simulink model "Tester_GX"  (R2026a)
settings: Solver=VariableStepAuto  StopTime=inf
libraries: instrumentlib x2, dspstat3 x1, dspindex x1, realtime_pacer_lib x1, simulink x1, slpidlib x1, SignalEditorBlockLib x1
settings Model: Creator=errikos  LastModifiedBy=hardik-karan
settings SimscapeCC: SimscapeNominalValues="[{\"value\":\"1\",\"unit\":\"A\"},{\"value\":\"1\",\"unit\":\"bar\"},{\"value\":\"1\",\"unit\":\"cm^2\"},{\"value\":\"1\",\"unit\":\"cm^3/s\"},{\"value\":\"1\",\"unit\":\"kJ/kg\"},{\"value\":\"1\",\"unit\":\"kW\"},{\"value\":\"1\",\"unit\":\"l\"},{\"value\":\"1\",\"unit\":\"N\"},{\"value\":\"1\",\"unit\":\"N*m\"},{\"value\":\"1\",\"unit\":\"V\"}]"  SimscapeLogType=none  SimscapeLogDecimation=1  SimscapeLogDataHistory=5000

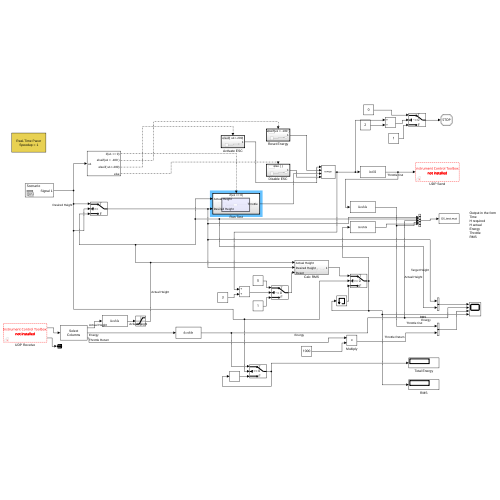
[thumbnail: Simulink's stored preview of the top-level diagram]
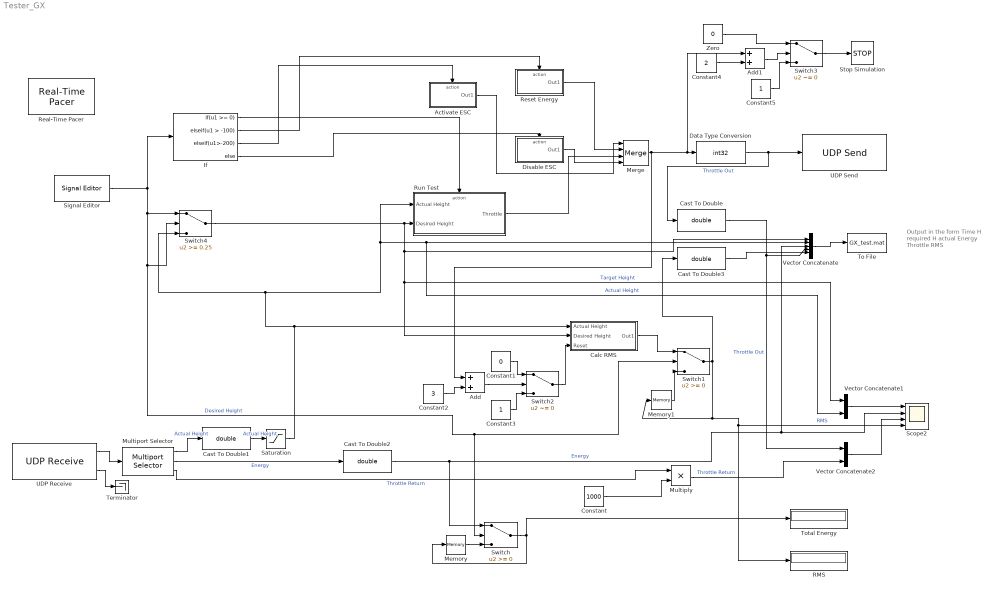
== system Tester_GX ==
  note: Output in the form
      | Time
      | H required
      | H actual
      | Energy
      | Throttle
      | RMS
  Activate ESC : Subsystem  TreatAsAtomicUnit=on
  Add : Sum
  Add1 : Sum
  Calc RMS : Subsystem
  Cast To Double{,1..3} (4 alike) : DataTypeConversion  OutDataTypeStr=double  SaturateOnIntegerOverflow=off  RndMeth=Floor
  Constant : Constant  Value=1000
  Constant1 : Constant  Value=0
  Constant2 : Constant  Value=3
  Constant3 : Constant
  Constant4 : Constant  Value=2
  Constant5 : Constant
  Data Type Conversion : DataTypeConversion  OutDataTypeStr=int32  SaturateOnIntegerOverflow=off  RndMeth=Floor
  Disable ESC : Subsystem  TreatAsAtomicUnit=on
  If : If  IfExpression=u1 >= 0  ElseIfExpressions=u1 > -100 , u1>-200
  Memory : Memory
  Memory1 : Memory
  Merge : Merge  Inputs=4
  Multiply : Product
  Multiport Selector : dspindex/Multiport Selector  rowsOrCols=Columns  idxCellArray={ 1, 2,3}  idxErrMode=Clip and Warn
  RMS : Display
  Real-Time Pacer : realtime_pacer_lib/Real-Time Pacer  simTimePerRealTime=1
  Reset Energy : Subsystem  TreatAsAtomicUnit=on
  Run Test : Subsystem  TreatAsAtomicUnit=on
  Saturation : Saturate  UpperLimit=1.7  LowerLimit=0
  Scope2 : Scope  NumInputPorts=4
      settings: TimeSpan=75  Title=Height  ActiveDisplayYMinimum=-0.02957  ActiveDisplayYMaximum=1.32226  YLabel=Height (m)  DataLoggingVariableName=ScopeData2
  Signal Editor : SignalEditorBlockLib/Signal Editor  FileName=/Users/errikoslevis/Downloads/Simulink Testing/samplemission.mat  ActiveScenario=Scenario  ActiveSignal=Signal 1  IsBus=off  OutputBusObjectStr=Bus: BusObject  SampleTime=0.05  ZeroCross=off  OutputAfterFinalValue=Setting to zero  Unit=inherit  PreserveSignalName=on  ApplySigPropsToAllScenarios=on  ApplySigPropsToAllSignals=off  SignalPropertySource=Dialog parameters
  Stop Simulation : Stop
  Switch : Switch  SaturateOnIntegerOverflow=off  InputSameDT=off
  Switch1 : Switch  SaturateOnIntegerOverflow=off  InputSameDT=off
  Switch2 : Switch  Criteria=u2 ~= 0  SaturateOnIntegerOverflow=off  InputSameDT=off
  Switch3 : Switch  Criteria=u2 ~= 0  ZeroCross=off  SaturateOnIntegerOverflow=off  InputSameDT=off
  Switch4 : Switch  Threshold=0.25  SaturateOnIntegerOverflow=off  InputSameDT=off
  Terminator : Terminator
  To File : ToFile  Filename=GX_test.mat
  Total Energy : Display
  UDP Receive : instrumentlib/UDP Receive  Host=192.168.0.110  Port=4000  LocalPort=8888  EnablePortSharing=on  GetLatestData=on  DataSize="[1  3]"  DataType=single  ASCIIFormatting=%f%f  Terminator=LF  ByteOrder=LittleEndian  EnableBlockingMode=off  Timeout=10  SampleTime=0.05  LocalAddress=192.168.0.100
  UDP Send : instrumentlib/UDP Send  Host=192.168.0.110  Port=4000  LocalPort=-1  EnablePortSharing=on  ByteOrder=LittleEndian  OutputDatagramPacketSize=4  EnableBlockingMode=on  LocalAddress=192.168.0.100
  Vector Concatenate : Concatenate  NumInputs=5
  Vector Concatenate1 : Concatenate
  Vector Concatenate2 : Concatenate
  Zero : Constant  Value=0  OutDataTypeStr=Inherit: Inherit via back propagation
  wires:
  UDP Receive/1 -> Multiport Selector/1
  Multiport Selector/1 -> Cast To Double1/1  "Actual Height"
  Multiport Selector/2 -> Cast To Double2/1  "Energy"
  Run Test/1("Throttle ") -> Merge/3
  Data Type Conversion/1 -> Cast To Double/1, UDP Send/1  "Throttle Out"
  Multiport Selector/3 -> Multiply/1  "Throttle Return"
  Multiply/1 -> Vector Concatenate2/2  "Throttle Return"
  Constant/1 -> Multiply/2
  Signal Editor/1 -> Switch4/2, Switch1/2, Switch/2, Switch4/1, If/1  "Desired Height"
  Merge/1 -> Add/1, Add1/1, Data Type Conversion/1
  Vector Concatenate/1 -> To File/1
  If/1 -> Run Test/Action
  If/2 -> Reset Energy/Action
  If/3 -> Activate ESC/Action
  If/4 -> Disable ESC/Action
  Activate ESC/1(Out1) -> Merge/1
  Disable ESC/1(Out1) -> Merge/4
  Switch/1 -> Memory/1, Total Energy/1
  Cast To Double/1 -> Vector Concatenate2/1, Vector Concatenate/4  "Throttle Out"
  Saturation/1 -> Switch4/3, Run Test/1(Actual Height), Vector Concatenate1/2, Vector Concatenate/2, Calc RMS/1(Actual Height)  "Actual Height"
  Cast To Double2/1 -> Switch/1, Scope2/2, Vector Concatenate/3  "Energy"
  Cast To Double3/1 -> Vector Concatenate/5
  Memory/1 -> Switch/3
  Switch1/1 -> RMS/1, Scope2/4, Memory1/1, Cast To Double3/1  "RMS"
  Memory1/1 -> Switch1/3
  Calc RMS/1(Out1) -> Switch1/1
  Switch2/1 -> Calc RMS/3(Reset)
  Constant1/1 -> Switch2/1
  Constant2/1 -> Add/2
  Add/1 -> Switch2/2
  Constant3/1 -> Switch2/3
  Reset Energy/1(Out1) -> Merge/2
  Switch3/1 -> Stop Simulation/1
  Zero/1 -> Switch3/1
  Add1/1 -> Switch3/2
  Constant4/1 -> Add1/2
  Constant5/1 -> Switch3/3
  Vector Concatenate2/1 -> Scope2/3
  Vector Concatenate1/1 -> Scope2/1
  Switch4/1 -> Vector Concatenate/1, Vector Concatenate1/1, Calc RMS/2(Desired Height), Run Test/2(Desired Height)  "Target Height"
  Cast To Double1/1 -> Saturation/1  "Actual Height"
  UDP Receive/2 -> Terminator/1

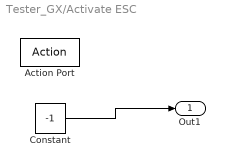
== system Tester_GX/Activate ESC ==
  Action Port : ActionPort  ActionPortLabel=elseif( u1>-200)
  Constant : Constant  Value=-1  SampleTime=0.05
  Out1 : Outport  VectorParamsAs1DForOutWhenUnconnected=off
  wires:
  Constant/1 -> Out1/1

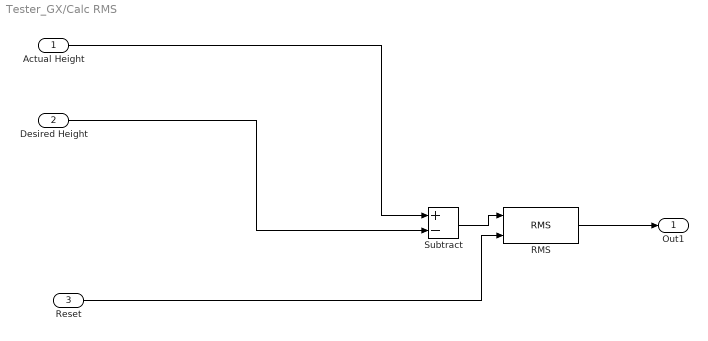
== system Tester_GX/Calc RMS ==
  Actual Height : Inport
  Desired Height : Inport  Port=2
  Reset : Inport  Port=3
  RMS : dspstat3/RMS  run=on  directionMode=Each column  dimension=1  reset_popup=Non-zero sample
  Subtract : Sum  Inputs=+-
  Out1 : Outport  VectorParamsAs1DForOutWhenUnconnected=off
  wires:
  Desired Height/1 -> Subtract/2
  Actual Height/1 -> Subtract/1
  RMS/1 -> Out1/1
  Subtract/1 -> RMS/1
  Reset/1 -> RMS/2

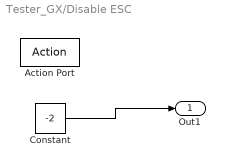
== system Tester_GX/Disable ESC ==
  Action Port : ActionPort  ActionPortLabel=else
  Constant : Constant  Value=-2  SampleTime=0.05
  Out1 : Outport  VectorParamsAs1DForOutWhenUnconnected=off
  wires:
  Constant/1 -> Out1/1

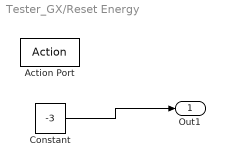
== system Tester_GX/Reset Energy ==
  Action Port : ActionPort  ActionPortLabel=elseif(u1 > -100 )
  Constant : Constant  Value=-3  SampleTime=0.05
  Out1 : Outport  VectorParamsAs1DForOutWhenUnconnected=off
  wires:
  Constant/1 -> Out1/1

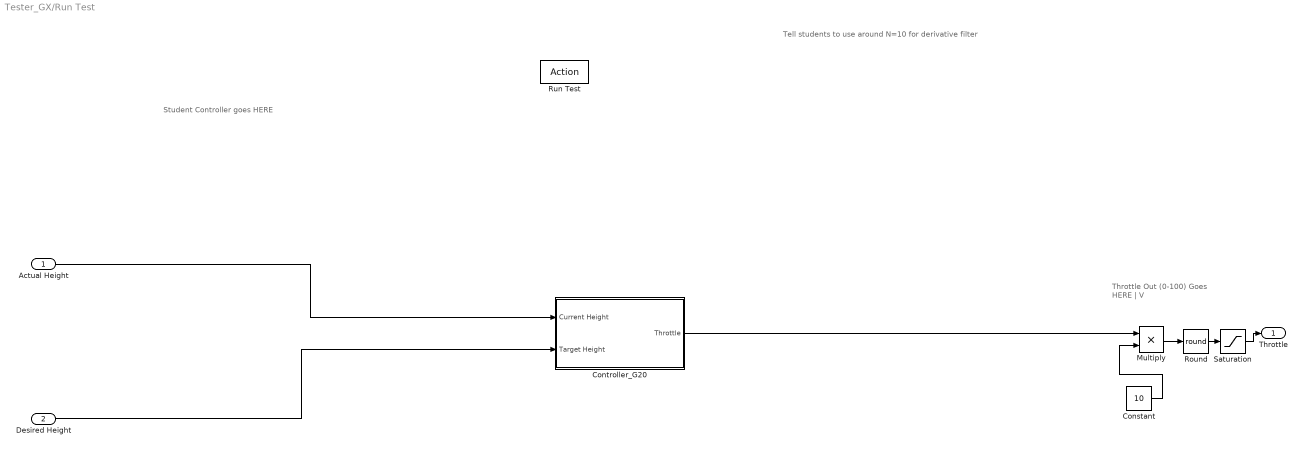
== system Tester_GX/Run Test ==
  note: Tell students to use around N=10 for derivative filter
  note: Throttle Out (0-100)
      | Goes HERE
      |            |
      | 	   V
  note: Student Controller goes HERE
  Actual Height : Inport
  Desired Height : Inport  Port=2
  Run Test : ActionPort  ActionPortLabel=if(u1 >= 0)
  Constant : Constant  Value=10
  Controller_G20 : Subsystem
  Multiply : Product
  Round : Rounding  Operator=round
  Saturation : Saturate  UpperLimit=1000  LowerLimit=0
  "Throttle " : Outport  VectorParamsAs1DForOutWhenUnconnected=off
  wires:
  Saturation/1 -> "Throttle "/1
  Constant/1 -> Multiply/2
  Multiply/1 -> Round/1
  Round/1 -> Saturation/1
  Desired Height/1 -> Controller_G20/2(Target Height)
  Actual Height/1 -> Controller_G20/1(Current Height)
  Controller_G20/1(Throttle) -> Multiply/1

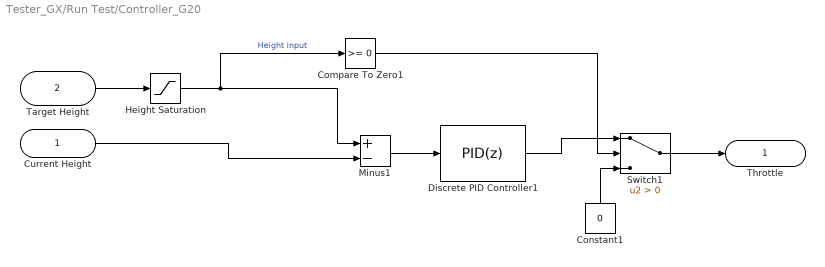
== system Tester_GX/Run Test/Controller_G20 ==
  Current Height : Inport
  Target Height : Inport  Port=2
  Compare To Zero1 : simulink/Logic and Bit Operations/Compare To Zero  relop=>=  OutDataTypeStr=boolean
  Constant1 : Constant  Value=0
  Discrete PID Controller1 : slpidlib/PID Controller  Controller=PID  Form=Parallel  TimeDomain=Discrete-time  UseExternalTs=off  SampleTime=-1  IntegratorMethod=Forward Euler  FilterMethod=Forward Euler  ControllerParametersSource=internal  P=81.87  I=187.7  UseKiTs=off  D=24.93  UseExternalDerivativeSource=off  N=8.97  UseFilter=on  TunerSelectOption=Frequency Response Based  InitialConditionSource=internal  InitialConditionForIntegrator=0  InitialConditionForFilter=0  DifferentiatorICPrevScaledInput=0  ExternalReset=none  TrackingMode=off  Kt=1  LimitOutput=on  SatLimitsSource=internal  UpperSaturationLimit=78  LowerSaturationLimit=0  LinearizeAsGain=off  AntiWindupMode=back-calculation  Kb=0.45  LimitIntegrator=off  UpperIntegratorSaturationLimit=inf  LowerIntegratorSaturationLimit=-inf  POutMin=[]  POutMax=[]  IOutMin=[]  IOutMax=[]  DOutMin=[]  DOutMax=[]  NOutMin=[]  NOutMax=[]  SumOutMin=[]  SumOutMax=[]  SaturationOutMin=[]  SaturationOutMax=[]  PParamMin=[]  PParamMax=[]  IParamMin=[]  IParamMax=[]  DParamMin=[]  DParamMax=[]  NParamMin=[]  NParamMax=[]  KbParamMin=[]  KbParamMax=[]  KtParamMin=[]  KtParamMax=[]  KbOutMin=[]  KbOutMax=[]  KtOutMin=[]  KtOutMax=[]  IntegratorOutMin=[]  IntegratorOutMax=[]  FilterOutMin=[]  FilterOutMax=[]  SumI1OutMin=[]  SumI1OutMax=[]  SumI2OutMin=[]  SumI2OutMax=[]  SumI3OutMin=[]  SumI3OutMax=[]  SumI4OutMin=[]  SumI4OutMax=[]  SumDOutMin=[]  SumDOutMax=[]  DifferentiatorOutMin=[]  DifferentiatorOutMax=[]  FilterDiffOutCoefMin=[]  FilterDiffOutCoefMax=[]  ReciprocalOutMin=[]  ReciprocalOutMax=[]  SumDenOutMin=[]  SumDenOutMax=[]  SumNumOutMin=[]  SumNumOutMax=[]  DivideOutMin=[]  DivideOutMax=[]  UdiffTsProdOutMin=[]  UdiffTsProdOutMax=[]  NTsProdOutMin=[]  NTsProdOutMax=[]  UintegralTsProdOutMin=[]  UintegralTsProdOutMax=[]  UngainTsProdOutMin=[]  UngainTsProdOutMax=[]  ClampingZeroOutDataTypeStr=Inherit: Inherit via back propagation  ClampingZeroOutMin=[]  ClampingZeroOutMax=[]  FilterDenConstantOutDataTypeStr=Inherit: Inherit via back propagation  FilterDenConstantOutMin=[]  FilterDenConstantOutMax=[]  PCopyOutDataTypeStr=Inherit: Inherit via back propagation  PCopyOutMin=[]  PCopyOutMax=[]  NCopyOutDataTypeStr=Inherit: Inherit via back propagation  NCopyOutMin=[]  NCopyOutMax=[]  IntegratorContinuousStateAttributes=''  IntegratorStateMustResolveToSignalObject=off  IntegratorRTWStateStorageClass=Auto  FilterContinuousStateAttributes=''  FilterStateMustResolveToSignalObject=off  FilterRTWStateStorageClass=Auto  ParallelPVariant=InternalParameters  IdealPVariant=Disabled  IVariant=InternalParameters  DVariant=InternalParameters  IntegratorVariant=Discrete  SatVariant=Enabled  AWVariant=BackCalculation  PCopyVariant=Disabled  TRVariant=Disabled  FdbkBlocksVariant=Forward  IdealPFdbkVariant=Disabled  SatFdbkVariant=Disabled  DerivativeFilterVariant=ForwardEulerFilter  NVariant=InternalParameters  NCopyVariant=Disabled  FilterICVariant=InternalICsFilter  IntegratorICVariant=InternalICs  ExternalResetVariant=Disabled  TRSumVariant=Passthrough  SumFdbkVariant=Disabled  SumVariant=Sum_PID  TsampFilterVariant=InternalTs  TsampNgainVariant=Passthrough  TsampIntegralVariant=Disabled_SignalSpec  ExternalSaturationOutDataTypeStr=Inherit: Same as second input  DerivativeSourceVariant=ErrorSignal  PreIntVariant=InternalPreInt
      settings: LibrarySourceBlock=simulink/Discrete/Discrete PID Controller
  Height Saturation : Saturate  UpperLimit=1.44  LowerLimit=0
  Minus1 : Sum  Inputs=+-
  Switch1 : Switch  Criteria=u2 > Threshold  SaturateOnIntegerOverflow=off  InputSameDT=off
  Throttle : Outport
  wires:
  Discrete PID Controller1/1 -> Switch1/1
  Target Height/1 -> Height Saturation/1
  Height Saturation/1 -> Minus1/1, Compare To Zero1/1  "Height input"
  Current Height/1 -> Minus1/2
  Minus1/1 -> Discrete PID Controller1/1
  Constant1/1 -> Switch1/3
  Switch1/1 -> Throttle/1
  Compare To Zero1/1 -> Switch1/2
